simulink model "without_sesnor_PID"  (R2015a)
settings: Solver=ode45  StartTime=0.0  StopTime=10.0  RelTol=1e-3
settings Model: Creator=Manoj  LastModifiedBy=Manoj

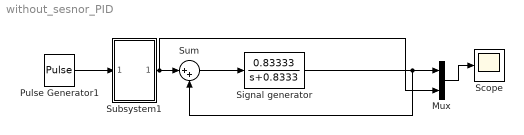
== system without_sesnor_PID ==
  Mux : Mux  Inputs=2
  Pulse Generator1 : DiscretePulseGenerator  PulseType=Time based  Period=4  PhaseDelay=0-1
  Scope : Scope
      settings: TimeRange=10  YMin=-0.004  YMax=0.008
  Signal generator : TransferFcn  Numerator=[0.83333]  Denominator=[1 0.8333]
  Subsystem1 : Subsystem
  Sum : Sum  Inputs=|++
  wires:
  Subsystem1/1(Out1) -> Mux/2, Sum/1
  Signal generator/1 -> Mux/1, Sum/2
  Pulse Generator1/1 -> Subsystem1/1(In1)
  Sum/1 -> Signal generator/1
  Mux/1 -> Scope/1

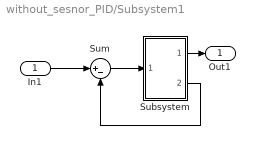
== system without_sesnor_PID/Subsystem1 ==
  In1 : Inport
  Subsystem : Subsystem
  Sum : Sum  Inputs=|+-
  Out1 : Outport
  wires:
  In1/1 -> Sum/1
  Subsystem/1(Out1) -> Out1/1
  Subsystem/2(Out2) -> Sum/2
  Sum/1 -> Subsystem/1(In1)

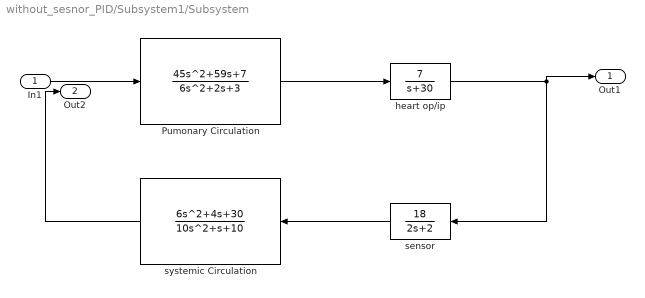
== system without_sesnor_PID/Subsystem1/Subsystem ==
  In1 : Inport
  Pumonary Circulation : TransferFcn  Numerator=[45 59 7]  Denominator=[6 2 3]
  heart op/ip : TransferFcn  Numerator=[7]  Denominator=[1 30]
  sensor : TransferFcn  Numerator=[18]  Denominator=[2 2]
  systemic Circulation : TransferFcn  Numerator=[6 4 30]  Denominator=[10 1 10]
  Out1 : Outport
  Out2 : Outport  Port=2
  wires:
  In1/1 -> Pumonary Circulation/1
  sensor/1 -> systemic Circulation/1
  heart op/ip/1 -> Out1/1, sensor/1
  systemic Circulation/1 -> Out2/1
  Pumonary Circulation/1 -> heart op/ip/1
